simulink model "WaermepumpeGrundlageIch"  (R2013a)
settings: Solver=ode4  StartTime=0.0  StopTime=inf  RelTol=1e-3
libraries: Thermolib x74, simulink x2
(part 2 of 2)

== system WaermepumpeGrundlageIch/Resorber/Heat Exchange/first media ==
  Qp : Inport
  FB1_in : Inport  Port=2
  Bus Assignment : BusAssignment  AssignedSignals=Hdot
  Bus Selector : BusSelector  OutputSignals=Hdot
  H-p-State with HeatLoss : Thermolib/Thermodynamic States and Properties/H-p-State with Heat Exchange  k=k_env  A_total=A_env/4  T_env=T_env  relaxation_factor=0.01  conv_limit=TH_THERM_H_P_STATE_T_CONV_LIMIT  hm_conv_limit=TH_THERM_H_P_STATE_HM_CONV_LIMIT  n_iteration=TH_THERM_H_P_STATE_NUM_ITER_MAX  T_initial=T_initial  H_initial=0  ndot_zero_eps=TH_THERM_NDOT_MIN
  Sum7 : Sum  Inputs=2  SaturateOnIntegerOverflow=on  InputSameDT=on  OutDataTypeStr=Inherit: Same as first input
  Terminator4 : Terminator
  FB1_out : Outport
  Q_env : Outport  Port=2
  wires:
  H-p-State with HeatLoss/3 -> Terminator4/1
  FB1_in/1 -> Bus Selector/1, Bus Assignment/1
  Qp/1 -> Sum7/1
  Sum7/1 -> Bus Assignment/2
  Bus Selector/1 -> Sum7/2  "<Hdot>"
  H-p-State with HeatLoss/1 -> FB1_out/1
  H-p-State with HeatLoss/2 -> Q_env/1
  Bus Assignment/1 -> H-p-State with HeatLoss/1

== system WaermepumpeGrundlageIch/Resorber/Heat Exchange/second media ==
  Qp : Inport
  FB2_in : Inport  Port=2
  Bus Assignment : BusAssignment  AssignedSignals=Hdot
  Bus Selector : BusSelector  OutputSignals=Hdot
  H-p-State with HeatLoss1 : Thermolib/Thermodynamic States and Properties/H-p-State with Heat Exchange  k=k_env  A_total=A_env/4  T_env=T_env  relaxation_factor=0.01  conv_limit=TH_THERM_H_P_STATE_T_CONV_LIMIT  hm_conv_limit=TH_THERM_H_P_STATE_HM_CONV_LIMIT  n_iteration=TH_THERM_H_P_STATE_NUM_ITER_MAX  T_initial=T_initial  H_initial=0  ndot_zero_eps=TH_THERM_NDOT_MIN
  Sum1 : Sum  Inputs=2  SaturateOnIntegerOverflow=on  InputSameDT=on  OutDataTypeStr=Inherit: Same as first input
  Terminator4 : Terminator
  FB2_out : Outport
  Q_env : Outport  Port=2
  wires:
  H-p-State with HeatLoss1/3 -> Terminator4/1
  H-p-State with HeatLoss1/1 -> FB2_out/1
  Sum1/1 -> Bus Assignment/2
  Qp/1 -> Sum1/1
  FB2_in/1 -> Bus Selector/1, Bus Assignment/1
  H-p-State with HeatLoss1/2 -> Q_env/1
  Bus Assignment/1 -> H-p-State with HeatLoss1/1
  Bus Selector/1 -> Sum1/2  "<Hdot>"

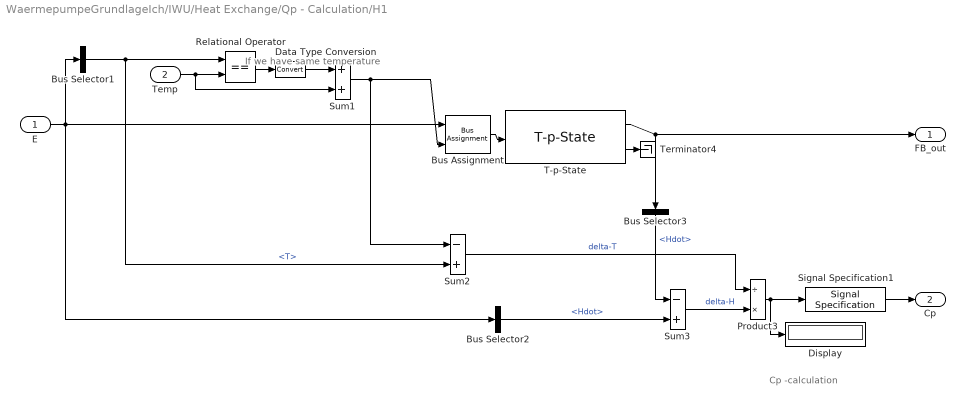
== system WaermepumpeGrundlageIch/IWU/Heat Exchange/Qp - Calculation/H1 ==
  note: If we have same temperature
  note: Cp -calculation
  E : Inport
  Temp : Inport  Port=2
  Bus Assignment : BusAssignment  AssignedSignals=T
  Bus Selector1 : BusSelector  OutputSignals=T
  Bus Selector2 : BusSelector  OutputSignals=Hdot
  Bus Selector3 : BusSelector  OutputSignals=Hdot
  Data Type Conversion : DataTypeConversion
  Display : Display
  Product3 : Product  Inputs=/*  SaturateOnIntegerOverflow=on  InputSameDT=on  OutDataTypeStr=Inherit: Same as first input
  Relational Operator : RelationalOperator  Operator===  OutDataTypeStr=boolean
  Signal Specification1 : SignalSpecification  Dimensions=1
  Sum1 : Sum  Inputs=2  SaturateOnIntegerOverflow=on  InputSameDT=on  OutDataTypeStr=Inherit: Same as first input
  Sum2 : Sum  Inputs=-+  SaturateOnIntegerOverflow=on  InputSameDT=on  OutDataTypeStr=Inherit: Same as first input
  Sum3 : Sum  Inputs=-+  SaturateOnIntegerOverflow=on  InputSameDT=on  OutDataTypeStr=Inherit: Same as first input
  T-p-State : Thermolib/Thermodynamic States and Properties/T-p-State
  Terminator4 : Terminator
  FB_out : Outport
  Cp : Outport  Port=2
  wires:
  Signal Specification1/1 -> Cp/1
  Bus Selector3/1 -> Sum3/1  "<Hdot>"
  Bus Selector2/1 -> Sum3/2  "<Hdot>"
  Product3/1 -> Signal Specification1/1, Display/1
  Sum2/1 -> Product3/1  "delta-T"
  Sum3/1 -> Product3/2  "delta-H"
  Data Type Conversion/1 -> Sum1/1
  Relational Operator/1 -> Data Type Conversion/1
  Temp/1 -> Sum1/2, Relational Operator/2
  E/1 -> Bus Assignment/1, Bus Selector2/1, Bus Selector1/1
  T-p-State/1 -> Bus Selector3/1, FB_out/1
  Bus Assignment/1 -> T-p-State/1
  Bus Selector1/1 -> Sum2/2, Relational Operator/1  "<T>"
  Sum1/1 -> Sum2/1, Bus Assignment/2
  T-p-State/2 -> Terminator4/1

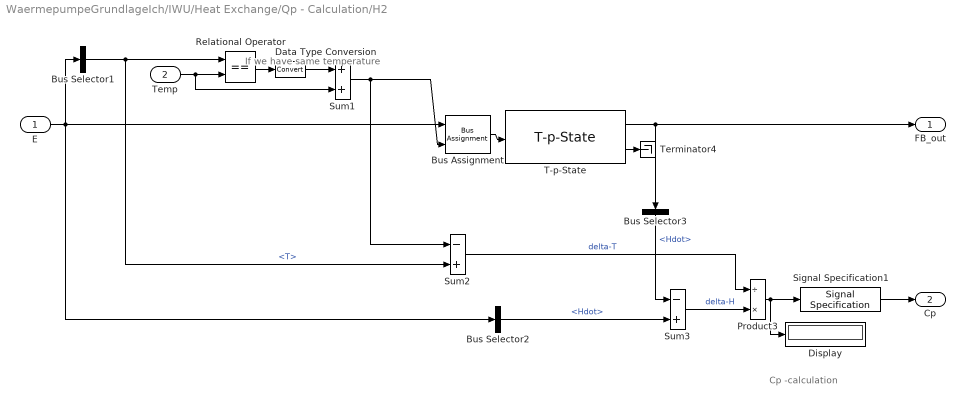
== system WaermepumpeGrundlageIch/IWU/Heat Exchange/Qp - Calculation/H2 ==
  note: Cp -calculation
  note: If we have same temperature
  E : Inport
  Temp : Inport  Port=2
  Bus Assignment : BusAssignment  AssignedSignals=T
  Bus Selector1 : BusSelector  OutputSignals=T
  Bus Selector2 : BusSelector  OutputSignals=Hdot
  Bus Selector3 : BusSelector  OutputSignals=Hdot
  Data Type Conversion : DataTypeConversion
  Display : Display
  Product3 : Product  Inputs=/*  SaturateOnIntegerOverflow=on  InputSameDT=on  OutDataTypeStr=Inherit: Same as first input
  Relational Operator : RelationalOperator  Operator===  OutDataTypeStr=boolean
  Signal Specification1 : SignalSpecification  Dimensions=1
  Sum1 : Sum  Inputs=2  SaturateOnIntegerOverflow=on  InputSameDT=on  OutDataTypeStr=Inherit: Same as first input
  Sum2 : Sum  Inputs=-+  SaturateOnIntegerOverflow=on  InputSameDT=on  OutDataTypeStr=Inherit: Same as first input
  Sum3 : Sum  Inputs=-+  SaturateOnIntegerOverflow=on  InputSameDT=on  OutDataTypeStr=Inherit: Same as first input
  T-p-State : Thermolib/Thermodynamic States and Properties/T-p-State
  Terminator4 : Terminator
  FB_out : Outport
  Cp : Outport  Port=2
  wires:
  Signal Specification1/1 -> Cp/1
  Sum1/1 -> Bus Assignment/2, Sum2/1
  Bus Selector1/1 -> Relational Operator/1, Sum2/2  "<T>"
  Bus Assignment/1 -> T-p-State/1
  T-p-State/1 -> FB_out/1, Bus Selector3/1
  E/1 -> Bus Selector1/1, Bus Selector2/1, Bus Assignment/1
  Temp/1 -> Relational Operator/2, Sum1/2
  Relational Operator/1 -> Data Type Conversion/1
  Data Type Conversion/1 -> Sum1/1
  Sum3/1 -> Product3/2  "delta-H"
  Sum2/1 -> Product3/1  "delta-T"
  Product3/1 -> Signal Specification1/1, Display/1
  Bus Selector2/1 -> Sum3/2  "<Hdot>"
  Bus Selector3/1 -> Sum3/1  "<Hdot>"
  T-p-State/2 -> Terminator4/1

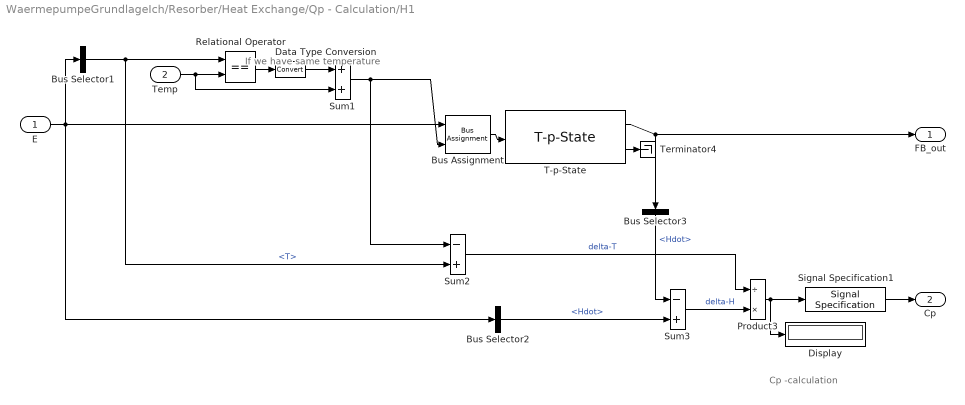
== system WaermepumpeGrundlageIch/Resorber/Heat Exchange/Qp - Calculation/H1 ==
  note: Cp -calculation
  note: If we have same temperature
  E : Inport
  Temp : Inport  Port=2
  Bus Assignment : BusAssignment  AssignedSignals=T
  Bus Selector1 : BusSelector  OutputSignals=T
  Bus Selector2 : BusSelector  OutputSignals=Hdot
  Bus Selector3 : BusSelector  OutputSignals=Hdot
  Data Type Conversion : DataTypeConversion
  Display : Display
  Product3 : Product  Inputs=/*  SaturateOnIntegerOverflow=on  InputSameDT=on  OutDataTypeStr=Inherit: Same as first input
  Relational Operator : RelationalOperator  Operator===  OutDataTypeStr=boolean
  Signal Specification1 : SignalSpecification  Dimensions=1
  Sum1 : Sum  Inputs=2  SaturateOnIntegerOverflow=on  InputSameDT=on  OutDataTypeStr=Inherit: Same as first input
  Sum2 : Sum  Inputs=-+  SaturateOnIntegerOverflow=on  InputSameDT=on  OutDataTypeStr=Inherit: Same as first input
  Sum3 : Sum  Inputs=-+  SaturateOnIntegerOverflow=on  InputSameDT=on  OutDataTypeStr=Inherit: Same as first input
  T-p-State : Thermolib/Thermodynamic States and Properties/T-p-State
  Terminator4 : Terminator
  FB_out : Outport
  Cp : Outport  Port=2
  wires:
  T-p-State/2 -> Terminator4/1
  Sum1/1 -> Bus Assignment/2, Sum2/1
  Bus Selector1/1 -> Relational Operator/1, Sum2/2  "<T>"
  Bus Assignment/1 -> T-p-State/1
  T-p-State/1 -> FB_out/1, Bus Selector3/1
  E/1 -> Bus Selector1/1, Bus Selector2/1, Bus Assignment/1
  Temp/1 -> Relational Operator/2, Sum1/2
  Relational Operator/1 -> Data Type Conversion/1
  Data Type Conversion/1 -> Sum1/1
  Sum3/1 -> Product3/2  "delta-H"
  Sum2/1 -> Product3/1  "delta-T"
  Product3/1 -> Display/1, Signal Specification1/1
  Bus Selector2/1 -> Sum3/2  "<Hdot>"
  Bus Selector3/1 -> Sum3/1  "<Hdot>"
  Signal Specification1/1 -> Cp/1

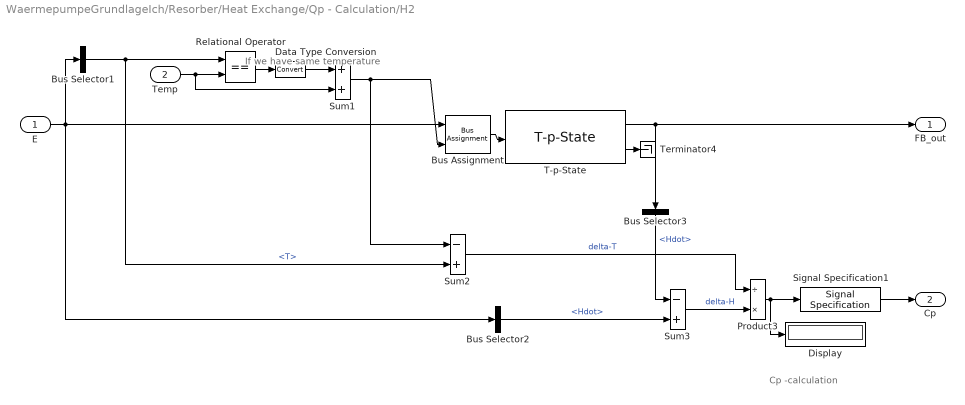
== system WaermepumpeGrundlageIch/Resorber/Heat Exchange/Qp - Calculation/H2 ==
  note: If we have same temperature
  note: Cp -calculation
  E : Inport
  Temp : Inport  Port=2
  Bus Assignment : BusAssignment  AssignedSignals=T
  Bus Selector1 : BusSelector  OutputSignals=T
  Bus Selector2 : BusSelector  OutputSignals=Hdot
  Bus Selector3 : BusSelector  OutputSignals=Hdot
  Data Type Conversion : DataTypeConversion
  Display : Display
  Product3 : Product  Inputs=/*  SaturateOnIntegerOverflow=on  InputSameDT=on  OutDataTypeStr=Inherit: Same as first input
  Relational Operator : RelationalOperator  Operator===  OutDataTypeStr=boolean
  Signal Specification1 : SignalSpecification  Dimensions=1
  Sum1 : Sum  Inputs=2  SaturateOnIntegerOverflow=on  InputSameDT=on  OutDataTypeStr=Inherit: Same as first input
  Sum2 : Sum  Inputs=-+  SaturateOnIntegerOverflow=on  InputSameDT=on  OutDataTypeStr=Inherit: Same as first input
  Sum3 : Sum  Inputs=-+  SaturateOnIntegerOverflow=on  InputSameDT=on  OutDataTypeStr=Inherit: Same as first input
  T-p-State : Thermolib/Thermodynamic States and Properties/T-p-State
  Terminator4 : Terminator
  FB_out : Outport
  Cp : Outport  Port=2
  wires:
  T-p-State/2 -> Terminator4/1
  Bus Selector3/1 -> Sum3/1  "<Hdot>"
  Bus Selector2/1 -> Sum3/2  "<Hdot>"
  Product3/1 -> Display/1, Signal Specification1/1
  Sum2/1 -> Product3/1  "delta-T"
  Sum3/1 -> Product3/2  "delta-H"
  Data Type Conversion/1 -> Sum1/1
  Relational Operator/1 -> Data Type Conversion/1
  Temp/1 -> Sum1/2, Relational Operator/2
  E/1 -> Bus Assignment/1, Bus Selector2/1, Bus Selector1/1
  T-p-State/1 -> Bus Selector3/1, FB_out/1
  Bus Assignment/1 -> T-p-State/1
  Bus Selector1/1 -> Sum2/2, Relational Operator/1  "<T>"
  Sum1/1 -> Sum2/1, Bus Assignment/2
  Signal Specification1/1 -> Cp/1
